simulink model "open_loop_system_obs"  (Simulink 7.7)
settings: Solver=ode45  StartTime=0.0  StopTime=10.0  RelTol=1e-3
values from neighbouring files (symbols this model uses):
  G = place((sys.a)', (sys.c(1,:))', Po)    [BE7_trame.m]
  Jt = 0.002    [BE7_trame.m]
  Kci = 1    [BE7_trame.m]
  Kcp = 1    [BE7_trame.m]
  Kcv = 0.0314    [BE7_trame.m]
  Ke = 0.2    [BE7_trame.m]
  Kg = 0.2    [BE7_trame.m]
  Le = 0.002    [BE7_trame.m]
  N = 300    [BE7_trame.m]
  Re = 2    [BE7_trame.m]
  sys = linmod('open_loop_system')    [BE7_trame.m]
libraries: simulink x2
settings Model: Creator=Anthony  LastModifiedBy=Anthony

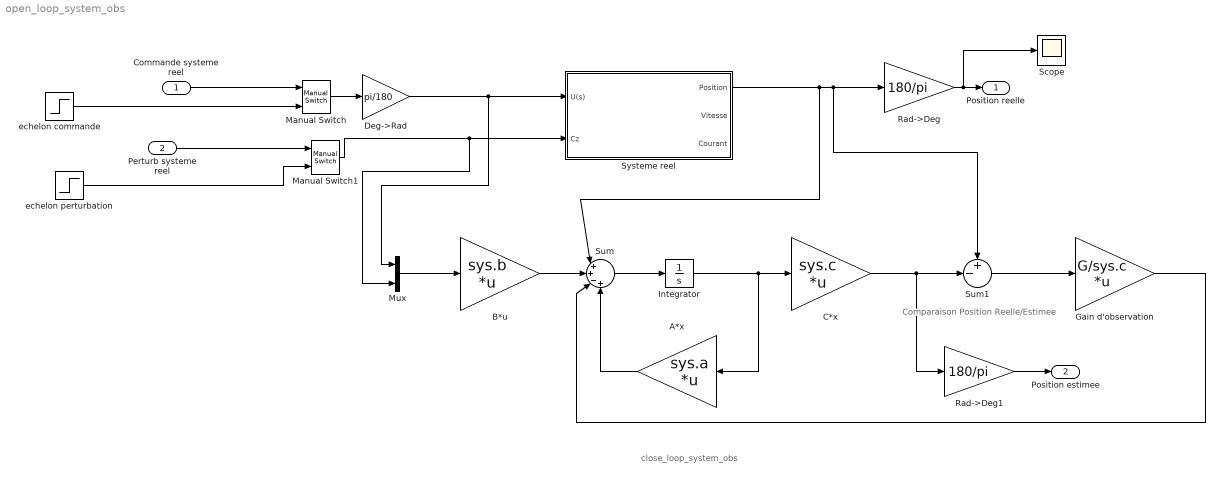
== system open_loop_system_obs ==
  note: close_loop_system_obs
  note: Comparaison Position
      | Reelle/Estimee
  Commande systeme reel : Inport
  Perturb systeme reel : Inport  Port=2
  A*x : Gain  Gain=sys.a  Multiplication=Matrix(K*u)
  B*u : Gain  Gain=sys.b  Multiplication=Matrix(K*u)
  C*x : Gain  Gain=sys.c  Multiplication=Matrix(K*u)
  Deg->Rad : Gain  Gain=pi/180
  Gain d'observation : Gain  Gain=G/sys.c  Multiplication=Matrix(K*u)
  Integrator : Integrator
  Manual Switch : simulink/Signal Routing/Manual Switch  SystemSampleTime=-1  sw=0  action=0  varsize=off
  Manual Switch1 : simulink/Signal Routing/Manual Switch  SystemSampleTime=-1  sw=0  action=0  varsize=off
  Mux : Mux  Inputs=2
  Rad->Deg : Gain  Gain=180/pi
  Rad->Deg1 : Gain  Gain=180/pi
  Scope : Scope
      settings: YMin=0.35  YMax=1.2
  Sum : Sum  Inputs=|++-+
  Sum1 : Sum  Inputs=+-|
  Systeme reel : Subsystem
  echelon commande : Step  Time=0  After=100  SampleTime=0
  echelon perturbation : Step  Time=5  After=0  SampleTime=0
  Position reelle : Outport
  Position estimee : Outport  Port=2
  wires:
  Systeme reel/1(Position) -> Sum/1, Rad->Deg/1, Sum1/1
  Integrator/1 -> C*x/1, A*x/1
  Sum/1 -> Integrator/1
  C*x/1 -> Sum1/2, Rad->Deg1/1
  Sum1/1 -> Gain d'observation/1
  Manual Switch1/1 -> Systeme reel/2(Cz), Mux/2
  Perturb systeme reel/1 -> Manual Switch1/1
  Commande systeme reel/1 -> Manual Switch/1
  echelon commande/1 -> Manual Switch/2
  echelon perturbation/1 -> Manual Switch1/2
  B*u/1 -> Sum/2
  A*x/1 -> Sum/4
  Gain d'observation/1 -> Sum/3
  Mux/1 -> B*u/1
  Manual Switch/1 -> Deg->Rad/1
  Deg->Rad/1 -> Systeme reel/1(U(s)), Mux/1
  Rad->Deg/1 -> Position reelle/1, Scope/1
  Rad->Deg1/1 -> Position estimee/1

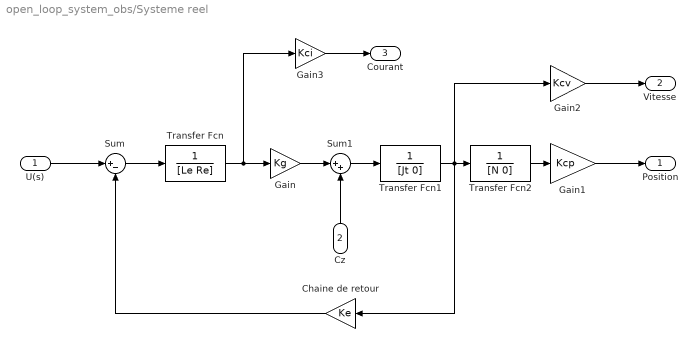
== system open_loop_system_obs/Systeme reel ==
  U(s) : Inport
  Cz : Inport  Port=2
  Chaine de retour : Gain  Gain=Ke
  Gain : Gain  Gain=Kg
  Gain1 : Gain  Gain=Kcp
  Gain2 : Gain  Gain=Kcv
  Gain3 : Gain  Gain=Kci
  Sum : Sum  Inputs=|+-
  Sum1 : Sum  Inputs=|++
  Transfer Fcn : TransferFcn  Denominator=[Le Re]
  Transfer Fcn1 : TransferFcn  Denominator=[Jt 0]
  Transfer Fcn2 : TransferFcn  Denominator=[N 0]
  Position : Outport
  Vitesse : Outport  Port=2
  Courant : Outport  Port=3
  wires:
  Gain1/1 -> Position/1
  Gain3/1 -> Courant/1
  Gain2/1 -> Vitesse/1
  Cz/1 -> Sum1/2
  U(s)/1 -> Sum/1
  Transfer Fcn2/1 -> Gain1/1
  Transfer Fcn1/1 -> Chaine de retour/1, Transfer Fcn2/1, Gain2/1
  Transfer Fcn/1 -> Gain/1, Gain3/1
  Sum/1 -> Transfer Fcn/1
  Sum1/1 -> Transfer Fcn1/1
  Gain/1 -> Sum1/1
  Chaine de retour/1 -> Sum/2
